simulink model "SW_8"  (R2013b)
settings: Solver=ode45  StartTime=0.0  StopTime=128  RelTol=1e-3
values from neighbouring files (symbols this model uses):
  const_val_lenqs = Nq-1    [confSim.m]    (also in preS_confSim.m)
  g = 1    [confSim.m]
  MiS = -5    [confSim.m]
  MS = 5    [confSim.m]
  nb_counter = ceil(log2(Ns))    [confSim.m]    (also in preS_confSim.m)
  NBitsScoreBus = 10    [confSim.m]    (also in preS_confSim.m)
  Nq = length(qCode)    [confSim.m]    (also in preS_confSim.m)
  Ns = length(sCode)    [confSim.m]    (also in preS_confSim.m)
  qCode = base2dec(q,Base)    [confSim.m]
  sCode = base2dec(s,Base)    [confSim.m]
  SMR_len = Nq*3    [confSim.m]    (also in preS_confSim.m)
libraries: xbsIndex_r4 x1212
(part 5 of 7)

== system SW_8/Subsystem/Subsystem5/P1_HW0 ==
  "reset " : Inport
  M_j-1(n)1 : Inport  Port=2
  MaxValue_j-1 : Inport  Port=3
  EndMaxRAM_j-1 : Inport  Port=4
  EndMaxP_j-1 : Inport  Port=5
  j-1 : Inport  Port=6
  s(n) : Inport  Port=7
  EnIn : Inport  Port=8
  q_j : Inport  Port=9
  AddSub : xbsIndex_r4/AddSub  mode=Addition  use_carryin=off  use_carryout=off  en=off  latency=as0  precision=User Defined  arith_type="Signed  (2's comp)"  n_bits=NBitsCalcInt  bin_pt=0  quantization=Truncate  overflow=Saturate  dbl_ovrd=off  use_behavioral_HDL=off  hw_selection=Fabric  pipelined=off  block_type=addsub
  AddSub1 : xbsIndex_r4/AddSub  mode=Subtraction  use_carryin=off  use_carryout=off  en=off  latency=as0  precision=User Defined  arith_type="Signed  (2's comp)"  n_bits=NBitsCalcInt  bin_pt=0  quantization=Truncate  overflow=Saturate  dbl_ovrd=off  use_behavioral_HDL=off  hw_selection=Fabric  pipelined=off  block_type=addsub
  AddSub2 : xbsIndex_r4/AddSub  mode=Subtraction  use_carryin=off  use_carryout=off  en=off  latency=as0  precision=User Defined  arith_type="Signed  (2's comp)"  n_bits=NBitsCalcInt  bin_pt=0  quantization=Truncate  overflow=Saturate  dbl_ovrd=off  use_behavioral_HDL=off  hw_selection=Fabric  pipelined=off  block_type=addsub
  Constant 0 : xbsIndex_r4/Constant  const=0  gui_display_data_type=Fixed-point  arith_type=Unsigned  n_bits=nb_bool  bin_pt=0  preci_type=Single  exp_width=8  frac_width=24  explicit_period=off  period=1  equ=P=C  opselect=C  inp2=PCIN>>17  opr=+  inp1=P  carry=CIN  dbl_ovrd=off  block_type=constant
  Convert : xbsIndex_r4/Convert  gui_display_data_type=Fixed-point  arith_type=Unsigned  n_bits=nb_bool  bin_pt=0  float_type=Single  exp_bits=8  fraction_bits=24  quantization=Truncate  overflow=Wrap  en=off  latency=c0  dbl_ovrd=off  pipeline=off  block_type=convert
  Convert1 : xbsIndex_r4/Convert  gui_display_data_type=Fixed-point  arith_type=Unsigned  n_bits=k  bin_pt=0  float_type=Single  exp_bits=8  fraction_bits=24  quantization=Truncate  overflow=Wrap  en=off  latency=c0  dbl_ovrd=off  pipeline=off  block_type=convert
  Convert2 : xbsIndex_r4/Convert  gui_display_data_type=Fixed-point  arith_type=Unsigned  n_bits=nb_bool  bin_pt=0  float_type=Single  exp_bits=8  fraction_bits=24  quantization=Truncate  overflow=Wrap  en=off  latency=c0  dbl_ovrd=off  pipeline=off  block_type=convert
  Convert3 : xbsIndex_r4/Convert  gui_display_data_type=Fixed-point  arith_type=Unsigned  n_bits=NBitsCalcInt  bin_pt=0  float_type=Single  exp_bits=8  fraction_bits=24  quantization=Truncate  overflow=Wrap  en=off  latency=c0  dbl_ovrd=off  pipeline=off  block_type=convert
  Convert4 : xbsIndex_r4/Convert  gui_display_data_type=Boolean  arith_type=Boolean  n_bits=1  bin_pt=0  float_type=Single  exp_bits=8  fraction_bits=24  quantization=Truncate  overflow=Wrap  en=off  latency=c0  dbl_ovrd=off  pipeline=off  block_type=convert
  Counter : xbsIndex_r4/Counter  cnt_type=Count Limited  cnt_to=counter_val  operation=Up  start_count=0  cnt_by_val=1  arith_type=Unsigned  n_bits=counter_num_b  bin_pt=0  load_pin=off  rst=on  en=on  explicit_period=on  period=Ts  dbl_ovrd=off  use_behavioral_HDL=off  implementation=Fabric  block_type=counter
  Inverter : xbsIndex_r4/Inverter  en=off  latency=l0  dbl_ovrd=off  block_type=inv
  Inverter1 : xbsIndex_r4/Inverter  en=off  latency=l0  dbl_ovrd=off  block_type=inv
  Inverter2 : xbsIndex_r4/Inverter  en=off  latency=l0  dbl_ovrd=off  block_type=inv
  Logical : xbsIndex_r4/Logical  logical_function=AND  inputs=2  en=off  latency=l0  precision=User Defined  arith_type=Unsigned  n_bits=nb_bool  bin_pt=0  align_bp=on  dbl_ovrd=off  block_type=logical
  MS Match_Score : xbsIndex_r4/Constant  const=MS  gui_display_data_type=Fixed-point  arith_type=Signed (2's comp)  n_bits=NBitsK  bin_pt=0  preci_type=Single  exp_width=8  frac_width=24  explicit_period=on  period=Ts  equ=P=C  opselect=C  inp2=PCIN>>17  opr=+  inp1=P  carry=CIN  dbl_ovrd=off  block_type=constant
  M_j(n-1) : xbsIndex_r4/Register  init=0  rst=on  en=on  dbl_ovrd=off  block_type=register
  Match and Mismtach Score : Subsystem
  Max1 : Subsystem
  MiS MisMatch_Score : xbsIndex_r4/Constant  const=MiS  gui_display_data_type=Fixed-point  arith_type=Signed (2's comp)  n_bits=NBitsK  bin_pt=0  preci_type=Single  exp_width=8  frac_width=24  explicit_period=on  period=Ts  equ=P=C  opselect=C  inp2=PCIN>>17  opr=+  inp1=P  carry=CIN  dbl_ovrd=off  block_type=constant
  Mux1 : xbsIndex_r4/Mux  inputs=2  en=off  latency=mft  precision=User Defined  arith_type=Unsigned  n_bits=counter_num_b  bin_pt=0  quantization=Truncate  overflow=Wrap  dbl_ovrd=off  block_type=mux
  Mux2 : xbsIndex_r4/Mux  inputs=2  en=off  latency=mft  precision=User Defined  arith_type=Unsigned  n_bits=NBitsCalcInt  bin_pt=0  quantization=Truncate  overflow=Wrap  dbl_ovrd=off  block_type=mux
  Mux3 : xbsIndex_r4/Mux  inputs=2  en=off  latency=mft  precision=User Defined  arith_type=Unsigned  n_bits=counter_num_b  bin_pt=0  quantization=Truncate  overflow=Wrap  dbl_ovrd=off  block_type=mux
  Mux4 : xbsIndex_r4/Mux  inputs=2  en=off  latency=mft  precision=User Defined  arith_type=Unsigned  n_bits=nb_lqC  bin_pt=0  quantization=Truncate  overflow=Wrap  dbl_ovrd=off  block_type=mux
  Mux5 : xbsIndex_r4/Mux  inputs=2  en=off  latency=mft  precision=User Defined  arith_type=Unsigned  n_bits=nb_bool  bin_pt=0  quantization=Truncate  overflow=Wrap  dbl_ovrd=off  block_type=mux
  Mux6 : xbsIndex_r4/Mux  inputs=2  en=off  latency=mft  precision=User Defined  arith_type=Unsigned  n_bits=NBitsCalcInt  bin_pt=0  quantization=Truncate  overflow=Wrap  dbl_ovrd=off  block_type=mux
  Mux7 : xbsIndex_r4/Mux  inputs=2  en=off  latency=mft  precision=User Defined  arith_type=Unsigned  n_bits=NBitsCalcInt  bin_pt=0  quantization=Truncate  overflow=Wrap  dbl_ovrd=off  block_type=mux
  Mux8 : xbsIndex_r4/Mux  inputs=2  en=off  latency=mft  precision=User Defined  arith_type=Unsigned  n_bits=k  bin_pt=0  quantization=Truncate  overflow=Wrap  dbl_ovrd=off  block_type=mux
  RM_j-1 : xbsIndex_r4/Register  init=0  rst=on  en=off  dbl_ovrd=off  block_type=register
  RM_j-2 : xbsIndex_r4/Register  init=0  rst=on  en=off  dbl_ovrd=off  block_type=register
  RMax_j : xbsIndex_r4/Register  init=0  rst=on  en=off  dbl_ovrd=off  block_type=register
  RMax_j2 : xbsIndex_r4/Register  init=0  rst=on  en=off  dbl_ovrd=off  block_type=register
  Relational1 : xbsIndex_r4/Relational  mode=a>b  en=off  latency=r0  dbl_ovrd=off  block_type=relational
  Relational2 : xbsIndex_r4/Relational  mode=a>b  en=off  latency=r0  dbl_ovrd=off  block_type=relational
  Relational3 : xbsIndex_r4/Relational  mode=a=b  en=off  latency=r0  dbl_ovrd=off  block_type=relational
  Relational4 : xbsIndex_r4/Relational  mode=a<b  en=off  latency=r0  dbl_ovrd=off  block_type=relational
  "bias " : xbsIndex_r4/Constant  const=1  gui_display_data_type=Fixed-point  arith_type=Signed (2's comp)  n_bits=NBitsScoreBus(1)  bin_pt=0  preci_type=Single  exp_width=8  frac_width=24  explicit_period=off  period=1  equ=P=C  opselect=C  inp2=PCIN>>17  opr=+  inp1=P  carry=CIN  dbl_ovrd=off  block_type=constant
  delay_sync{2,4,9..10} (4 alike) : xbsIndex_r4/Register  init=0  rst=on  en=off  dbl_ovrd=off  block_type=register
  delay_sync8 : xbsIndex_r4/Register  init=0  rst=off  en=off  dbl_ovrd=off  block_type=register
  g Gap_Penalty : xbsIndex_r4/Constant  const=g  gui_display_data_type=Fixed-point  arith_type=Signed (2's comp)  n_bits=NBitsK  bin_pt=0  preci_type=Single  exp_width=8  frac_width=24  explicit_period=on  period=Ts  equ=P=C  opselect=C  inp2=PCIN>>17  opr=+  inp1=P  carry=CIN  dbl_ovrd=off  block_type=constant
  len_q(s) Match_Score1 : xbsIndex_r4/Constant  const=const_val_lenqs  gui_display_data_type=Fixed-point  arith_type=Unsigned  n_bits=const_num_b_lenqs  bin_pt=0  preci_type=Single  exp_width=8  frac_width=24  explicit_period=off  period=1  equ=P=C  opselect=C  inp2=PCIN>>17  opr=+  inp1=P  carry=CIN  dbl_ovrd=off  block_type=constant
  "u+bias " : xbsIndex_r4/AddSub  mode=Addition  use_carryin=off  use_carryout=off  en=off  latency=0  precision=User Defined  arith_type="Signed  (2's comp)"  n_bits=NBitsCalcInt  bin_pt=0  quantization=Truncate  overflow=Saturate  dbl_ovrd=off  use_behavioral_HDL=off  hw_selection=Fabric  pipelined=off  block_type=addsub
  M_j(n) : Outport
  MaxValue : Outport  Port=2
  EndMaxRAM (valor de i) : Outport  Port=3
  EndMaxP (valor de j) : Outport  Port=4
  j : Outport  Port=5
  s(n-1) : Outport  Port=6
  EnOut(n) : Outport  Port=7
  Direction : Outport  Port=8
  wEnd : Outport  Port=9
  TraceBackStart : Outport  Port=10
  out_j : Outport  Port=11
  wires:
  Mux7/1 -> Relational1/1, Mux6/3, M_j(n)/1, M_j(n-1)/1
  Max1/2(value) -> Mux7/2
  Convert3/1 -> Mux7/3
  Convert1/1 -> Mux8/3
  Mux8/1 -> Direction/1
  Inverter2/1 -> Mux8/1
  Inverter1/1 -> Mux7/1
  Logical/1 -> Convert4/1
  Relational3/1 -> Mux5/1, Inverter/1
  j-1/1 -> out_j/1, Relational3/1, "u+bias "/1, Mux4/3
  delay_sync10/1 -> EnOut(n)/1
  delay_sync9/1 -> TraceBackStart/1
  q_j/1 -> Match and Mismtach Score/1(q_j)
  Relational4/1 -> Convert2/1
  Convert2/1 -> Mux5/3
  delay_sync8/1 -> Relational4/2
  Convert/1 -> Relational4/1, delay_sync8/1
  Inverter/1 -> Logical/2
  Constant 0/1 -> Mux5/2
  len_q(s) Match_Score1/1 -> Relational3/2
  Mux4/1 -> EndMaxP (valor de j)/1
  Mux3/1 -> EndMaxRAM (valor de i)/1
  Mux2/1 -> MaxValue/1
  MaxValue_j-1/1 -> Relational2/2, Mux2/2
  EndMaxRAM_j-1/1 -> Mux3/2
  EndMaxP_j-1/1 -> Mux4/2
  delay_sync4/1 -> j/1
  "u+bias "/1 -> delay_sync4/1
  "bias "/1 -> "u+bias "/2
  delay_sync2/1 -> s(n-1)/1
  Relational2/1 -> Mux2/1, Mux3/1, Mux4/1
  RMax_j2/1 -> Mux3/3, Mux1/2
  Mux1/1 -> RMax_j2/1
  RMax_j/1 -> Relational1/2, Relational2/1, Mux2/3, Mux6/2
  Relational1/1 -> Mux1/1, Mux6/1
  Mux6/1 -> RMax_j/1
  Counter/1 -> wEnd/1, Mux1/3
  Match and Mismtach Score/1(MS(q_j,s(n))) -> AddSub/1
  s(n)/1 -> Match and Mismtach Score/2(s(n)), delay_sync2/1  "s(n-1)"
  M_j(n-1)/1 -> AddSub2/1  "RM_j(n-1)"
  AddSub2/1 -> Max1/1((i-1,j))  "(i-1,j)"
  AddSub/1 -> Max1/3((i-1,j-1))  "(i-1,j-1)"
  AddSub1/1 -> Max1/2((i,j-1))  "(i,j-1)"
  g Gap_Penalty/1 -> AddSub2/2, AddSub1/2  "g"
  MiS MisMatch_Score/1 -> Match and Mismtach Score/4(MiS)
  MS Match_Score/1 -> Match and Mismtach Score/3(MS)
  RM_j-1/1 -> AddSub1/1, RM_j-2/1  "M_j-1(n-1)"
  M_j-1(n)1/1 -> RM_j-1/1
  RM_j-2/1 -> AddSub/2  "M_j-1(n-2)"
  Max1/1(ind) -> Mux8/2
  Convert4/1 -> delay_sync10/1
  Mux5/1 -> delay_sync9/1
  "reset "/1 -> delay_sync2/2, RM_j-1/2, delay_sync4/2, delay_sync10/2, delay_sync9/2, RMax_j/2, RMax_j2/2, M_j(n-1)/2, Counter/1, RM_j-2/2
  EnIn/1 -> Inverter2/1, Convert1/1, Inverter1/1, Convert3/1, M_j(n-1)/3, Counter/2, Convert/1, Logical/1

== system SW_8/Subsystem/Subsystem5/_RAM_0 ==
  En(n) : Inport
  RAM_j(n)=i : Inport  Port=2
  D_j(n) : Inport  Port=3
  BT_RAM_j(n)=i : Inport  Port=4
  BTRAMCont : Inport  Port=5
  Concat : xbsIndex_r4/Concat  num_inputs=2  dbl_ovrd=off  block_type=concat
  Logical3 : xbsIndex_r4/Logical  logical_function=AND  inputs=2  en=off  latency=l0  precision=User Defined  arith_type=Unsigned  n_bits=k  bin_pt=0  align_bp=on  dbl_ovrd=off  block_type=logical
  Mux3 : xbsIndex_r4/Mux  inputs=2  en=off  latency=mft  precision=User Defined  arith_type=Unsigned  n_bits=counter_num_b  bin_pt=0  quantization=Truncate  overflow=Wrap  dbl_ovrd=off  block_type=mux
  "RNq " : xbsIndex_r4/Register  init=0  rst=off  en=off  dbl_ovrd=off  block_type=register
  Register : xbsIndex_r4/Register  init=0  rst=off  en=off  dbl_ovrd=off  block_type=register
  Register2 : xbsIndex_r4/Register  init=0  rst=off  en=off  dbl_ovrd=off  block_type=register
  Register4 : xbsIndex_r4/Register  init=0  rst=off  en=off  dbl_ovrd=off  block_type=register
  SWBTRAM1 : xbsIndex_r4/Mux  inputs=2  en=off  latency=mft  precision=User Defined  arith_type=Unsigned  n_bits=nb_bool  bin_pt=0  quantization=Truncate  overflow=Wrap  dbl_ovrd=off  block_type=mux
  Single Port RAM2 : xbsIndex_r4/Single Port RAM  depth=length(sCode)  initVector=zeros(1,length(sCode))  distributed_mem=Distributed memory  write_mode=Read After Write  rst=off  init_reg=0  en=off  latency=Ts  dbl_ovrd=off  optimize=Area  block_type=spram
  D_j(n)1 : Outport
  wires:
  RAM_j(n)=i/1 -> Register2/1
  En(n)/1 -> Register/1
  D_j(n)/1 -> Register4/1
  SWBTRAM1/1 -> Concat/2, Concat/1
  "RNq "/1 -> Logical3/2
  Mux3/1 -> Single Port RAM2/1
  Single Port RAM2/1 -> Logical3/1
  Concat/1 -> "RNq "/1
  Register/1 -> SWBTRAM1/2, Single Port RAM2/3
  BT_RAM_j(n)=i/1 -> Mux3/3
  Register2/1 -> Mux3/2
  BTRAMCont/1 -> Mux3/1, SWBTRAM1/3, SWBTRAM1/1
  Register4/1 -> Single Port RAM2/2
  Logical3/1 -> D_j(n)1/1

== system SW_8/Subsystem/Subsystem5/seq_switch ==
  q_j(n) : Inport
  "Enable " : Inport  Port=2
  "reset " : Inport  Port=3
  Mux5 : xbsIndex_r4/Mux  inputs=2  en=off  latency=mft  precision=User Defined  arith_type=Unsigned  n_bits=k  bin_pt=0  quantization=Truncate  overflow=Wrap  dbl_ovrd=off  block_type=mux
  U>U/z : Subsystem
  delay_sync1 : xbsIndex_r4/Register  init=0  rst=on  en=off  dbl_ovrd=off  block_type=register
  q_j : Outport
  q_j(n-1) : Outport  Port=2
  wires:
  delay_sync1/1 -> Mux5/2
  U>U/z/1(Out1) -> Mux5/1
  Mux5/1 -> delay_sync1/1, q_j/1
  q_j(n)/1 -> Mux5/3, q_j(n-1)/1  "q_j(n-1)"
  "Enable "/1 -> U>U/z/1(In1)
  "reset "/1 -> delay_sync1/2, U>U/z/2(reset)

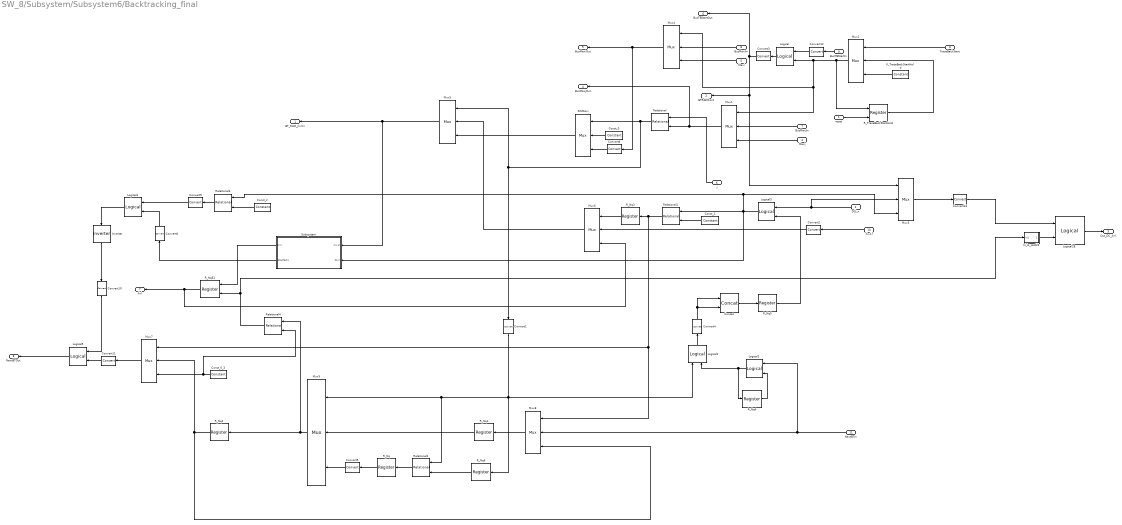
== system SW_8/Subsystem/Subsystem6/Backtracking_final ==
  "reset " : Inport
  "D(j)_n " : Inport  Port=2
  TraceBackStart : Inport  Port=3
  Maxj : Inport  Port=4
  Maxi : Inport  Port=5
  j : Inport  Port=6
  BusMaxjIn : Inport  Port=7
  BusMaxiIn : Inport  Port=8
  BusTBStartIn : Inport  Port=9
  i(n-1) : Inport  Port=10
  NextBTIn : Inport  Port=11
  Concat : xbsIndex_r4/Concat  num_inputs=2  dbl_ovrd=off  block_type=concat
  Const_0 : xbsIndex_r4/Constant  const=0  gui_display_data_type=Fixed-point  arith_type=Unsigned  n_bits=1  bin_pt=0  preci_type=Single  exp_width=8  frac_width=24  explicit_period=on  period=Ts  equ=P=C  opselect=C  inp2=PCIN>>17  opr=+  inp1=P  carry=CIN  dbl_ovrd=off  block_type=constant
  Const_0_3 : xbsIndex_r4/Constant  const=0  gui_display_data_type=Fixed-point  arith_type=Unsigned  n_bits=1  bin_pt=0  preci_type=Single  exp_width=8  frac_width=24  explicit_period=on  period=Ts  equ=P=C  opselect=C  inp2=PCIN>>17  opr=+  inp1=P  carry=CIN  dbl_ovrd=off  block_type=constant
  Const_1 : xbsIndex_r4/Constant  const=1  gui_display_data_type=Fixed-point  arith_type=Unsigned  n_bits=k  bin_pt=0  preci_type=Single  exp_width=8  frac_width=24  explicit_period=on  period=Ts  equ=P=C  opselect=C  inp2=PCIN>>17  opr=+  inp1=P  carry=CIN  dbl_ovrd=off  block_type=constant
  Const_2 : xbsIndex_r4/Constant  const=0  gui_display_data_type=Fixed-point  arith_type=Unsigned  n_bits=k  bin_pt=0  preci_type=Single  exp_width=8  frac_width=24  explicit_period=on  period=Ts  equ=P=C  opselect=C  inp2=PCIN>>17  opr=+  inp1=P  carry=CIN  dbl_ovrd=off  block_type=constant
  Convert1 : xbsIndex_r4/Convert  gui_display_data_type=Fixed-point  arith_type=Unsigned  n_bits=1  bin_pt=0  float_type=Single  exp_bits=8  fraction_bits=24  quantization=Truncate  overflow=Wrap  en=off  latency=c0  dbl_ovrd=off  pipeline=off  block_type=convert
  Convert{5,8..11} (5 alike) : xbsIndex_r4/Convert  gui_display_data_type=Fixed-point  arith_type=Unsigned  n_bits=nb_bool  bin_pt=0  float_type=Single  exp_bits=8  fraction_bits=24  quantization=Truncate  overflow=Wrap  en=off  latency=c0  dbl_ovrd=off  pipeline=off  block_type=convert
  Convert12 : xbsIndex_r4/Convert  gui_display_data_type=Fixed-point  arith_type=Unsigned  n_bits=1  bin_pt=0  float_type=Single  exp_bits=8  fraction_bits=24  quantization=Truncate  overflow=Wrap  en=off  latency=c0  dbl_ovrd=off  pipeline=off  block_type=convert
  Convert13 : xbsIndex_r4/Convert  gui_display_data_type=Fixed-point  arith_type=Unsigned  n_bits=k  bin_pt=0  float_type=Single  exp_bits=8  fraction_bits=24  quantization=Truncate  overflow=Wrap  en=off  latency=0  dbl_ovrd=off  pipeline=off  block_type=convert
  Convert2 : xbsIndex_r4/Convert  gui_display_data_type=Fixed-point  arith_type=Unsigned  n_bits=counter_num_b  bin_pt=0  float_type=Single  exp_bits=8  fraction_bits=24  quantization=Truncate  overflow=Wrap  en=off  latency=c0  dbl_ovrd=off  pipeline=off  block_type=convert
  Convert3 : xbsIndex_r4/Convert  gui_display_data_type=Boolean  arith_type=Boolean  n_bits=1  bin_pt=0  float_type=Single  exp_bits=8  fraction_bits=24  quantization=Truncate  overflow=Wrap  en=off  latency=c0  dbl_ovrd=off  pipeline=off  block_type=convert
  Convert4 : xbsIndex_r4/Convert  gui_display_data_type=Boolean  arith_type=Boolean  n_bits=1  bin_pt=0  float_type=Single  exp_bits=8  fraction_bits=24  quantization=Truncate  overflow=Wrap  en=off  latency=c0  dbl_ovrd=off  pipeline=off  block_type=convert
  Convert6 : xbsIndex_r4/Convert  gui_display_data_type=Fixed-point  arith_type=Unsigned  n_bits=counter_num_b  bin_pt=0  float_type=Single  exp_bits=8  fraction_bits=24  quantization=Truncate  overflow=Wrap  en=off  latency=c0  dbl_ovrd=off  pipeline=off  block_type=convert
  Inverter : xbsIndex_r4/Inverter  en=off  latency=l0  dbl_ovrd=off  block_type=inv
  K_TraceBackStartHold : xbsIndex_r4/Constant  const=1  gui_display_data_type=Fixed-point  arith_type=Unsigned  n_bits=1  bin_pt=0  preci_type=Single  exp_width=8  frac_width=24  explicit_period=on  period=Ts  equ=P=C  opselect=C  inp2=PCIN>>17  opr=+  inp1=P  carry=CIN  dbl_ovrd=off  block_type=constant
  Logical{,1..2,4} (4 alike) : xbsIndex_r4/Logical  logical_function=OR  inputs=2  en=off  latency=l0  precision=User Defined  arith_type=Unsigned  n_bits=nb_bool  bin_pt=0  align_bp=on  dbl_ovrd=off  block_type=logical
  Logical28 : xbsIndex_r4/Logical  logical_function=AND  inputs=2  en=off  latency=l0  precision=User Defined  arith_type=Unsigned  n_bits=k  bin_pt=0  align_bp=on  dbl_ovrd=off  block_type=logical
  Logical3 : xbsIndex_r4/Logical  logical_function=AND  inputs=2  en=off  latency=l0  precision=User Defined  arith_type=Unsigned  n_bits=k  bin_pt=0  align_bp=on  dbl_ovrd=off  block_type=logical
  Logical5 : xbsIndex_r4/Logical  logical_function=AND  inputs=2  en=off  latency=l0  precision=User Defined  arith_type=Unsigned  n_bits=nb_bool  bin_pt=0  align_bp=on  dbl_ovrd=off  block_type=logical
  Mux1 : xbsIndex_r4/Mux  inputs=2  en=off  latency=mft  precision=User Defined  arith_type=Unsigned  n_bits=nb_lqC  bin_pt=0  quantization=Truncate  overflow=Wrap  dbl_ovrd=off  block_type=mux
  Mux2 : xbsIndex_r4/Mux  inputs=2  en=off  latency=mft  precision=User Defined  arith_type=Unsigned  n_bits=nb_bool  bin_pt=0  quantization=Truncate  overflow=Wrap  dbl_ovrd=off  block_type=mux
  Mux3 : xbsIndex_r4/Mux  inputs=2  en=off  latency=mft  precision=User Defined  arith_type=Unsigned  n_bits=k  bin_pt=0  quantization=Truncate  overflow=Wrap  dbl_ovrd=off  block_type=mux
  Mux4 : xbsIndex_r4/Mux  inputs=2  en=off  latency=mft  precision=User Defined  arith_type=Unsigned  n_bits=counter_num_b  bin_pt=0  quantization=Truncate  overflow=Wrap  dbl_ovrd=off  block_type=mux
  Mux5 : xbsIndex_r4/Mux  inputs=2  en=off  latency=mft  precision=User Defined  arith_type=Unsigned  n_bits=counter_num_b  bin_pt=0  quantization=Truncate  overflow=Wrap  dbl_ovrd=off  block_type=mux
  Mux6 : xbsIndex_r4/Mux  inputs=2  en=off  latency=mft  precision=User Defined  arith_type=Unsigned  n_bits=counter_num_b  bin_pt=0  quantization=Truncate  overflow=Wrap  dbl_ovrd=off  block_type=mux
  Mux7 : xbsIndex_r4/Mux  inputs=2  en=off  latency=0  precision=User Defined  arith_type=Unsigned  n_bits=nb_bool  bin_pt=0  quantization=Truncate  overflow=Wrap  dbl_ovrd=off  block_type=mux
  Mux8 : xbsIndex_r4/Mux  inputs=2  en=off  latency=mft  precision=User Defined  arith_type=Unsigned  n_bits=nb_bool  bin_pt=0  quantization=Truncate  overflow=Wrap  dbl_ovrd=off  block_type=mux
  Mux9 : xbsIndex_r4/Mux  inputs=2  en=off  latency=mft  precision=User Defined  arith_type=Unsigned  n_bits=nb_bool  bin_pt=0  quantization=Truncate  overflow=Wrap  dbl_ovrd=off  block_type=mux
  R_Nq{,1..6} (7 alike) : xbsIndex_r4/Register  init=0  rst=off  en=off  dbl_ovrd=off  block_type=register
  R_NqE1 : xbsIndex_r4/Register  init=0  rst=off  en=on  dbl_ovrd=off  block_type=register
  R_TraceBackStartHold : xbsIndex_r4/Register  init=0  rst=on  en=off  dbl_ovrd=off  block_type=register
  Relational : xbsIndex_r4/Relational  mode=a=b  en=off  latency=r0  dbl_ovrd=off  block_type=relational
  Relational1 : xbsIndex_r4/Relational  mode=a=b  en=off  latency=r0  dbl_ovrd=off  block_type=relational
  Relational2 : xbsIndex_r4/Relational  mode=a>b  en=off  latency=r0  dbl_ovrd=off  block_type=relational
  Relational3 : xbsIndex_r4/Relational  mode=a=b  en=off  latency=0  dbl_ovrd=off  block_type=relational
  Relational4 : xbsIndex_r4/Relational  mode=a>b  en=off  latency=r0  dbl_ovrd=off  block_type=relational
  SWMaxi : xbsIndex_r4/Mux  inputs=2  en=off  latency=mft  precision=User Defined  arith_type=Unsigned  n_bits=counter_num_b  bin_pt=0  quantization=Truncate  overflow=Wrap  dbl_ovrd=off  block_type=mux
  Subsystem : Subsystem
  hi_lo_cast22 : Subsystem
  BT_RAM_j(n)=i : Outport
  BTRAMCont : Outport  Port=2
  Out_DC_j(n) : Outport  Port=3
  BusMaxjOut : Outport  Port=4
  BusMaxiOut : Outport  Port=5
  BusTBStartOut : Outport  Port=6
  i(n) : Outport  Port=7
  NextBTOut : Outport  Port=8
  wires:
  Logical28/1 -> Out_DC_j(n)/1
  hi_lo_cast22/1(Out1) -> Logical28/2
  Relational4/1 -> R_NqE1/2, hi_lo_cast22/1(In1)
  Convert13/1 -> Logical28/1
  Convert12/1 -> Logical/1
  Convert11/1 -> Logical5/2
  Convert10/1 -> Logical5/1
  Inverter/1 -> Convert10/1
  Mux7/1 -> Convert11/1
  Logical4/1 -> Inverter/1
  Subsystem/2(StopTBC1) -> Convert8/1
  Convert9/1 -> Logical4/1
  Convert8/1 -> Logical4/2
  Relational3/1 -> Convert9/1
  Const_2/1 -> Relational3/2
  Logical3/1 -> Relational1/1, Mux3/3, Relational3/1, Subsystem/2(D(n))
  Convert3/1 -> Mux3/1, BTRAMCont/1, BusTBStartOut/1
  Logical5/1 -> NextBTOut/1
  Mux4/1 -> Convert6/1, BusMaxiOut/1
  Mux1/1 -> Relational/2, BusMaxjOut/1
  R_NqE1/1 -> Mux6/3, i(n)/1
  Mux5/1 -> Subsystem/1(i(n-1)), BT_RAM_j(n)=i/1
  BusMaxjIn/1 -> Mux1/2
  Maxj/1 -> Mux1/3
  Maxi/1 -> Mux4/3
  TraceBackStart/1 -> Mux2/1
  j/1 -> Relational/1
  BusMaxiIn/1 -> Mux4/2
  BusTBStartIn/1 -> Convert12/1
  NextBTIn/1 -> Logical1/1, Mux8/2
  i(n-1)/1 -> Convert2/1
  "D(j)_n "/1 -> Logical3/1, Mux3/2
  Mux3/1 -> Convert13/1
  Mux2/1 -> R_TraceBackStartHold/1, Logical/2, Mux1/1, Mux4/1
  Convert6/1 -> SWMaxi/3
  SWMaxi/1 -> Mux5/3
  Mux6/1 -> Mux5/2
  Convert5/1 -> Mux9/3
  Mux9/1 -> Relational4/1, R_Nq2/1
  Convert2/1 -> Mux6/2
  Convert1/1 -> Mux9/1, Relational2/1, R_Nq6/1, Logical2/1
  Relational/1 -> SWMaxi/1, Convert1/1, Mux5/1
  Convert4/1 -> Concat/2, Concat/1
  R_Nq6/1 -> Relational2/2
  R_Nq1/1 -> Mux9/2
  R_Nq/1 -> Convert5/1
  R_TraceBackStartHold/1 -> Mux2/2
  Const_0/1 -> SWMaxi/2
  Mux8/1 -> R_Nq1/1
  Relational2/1 -> R_Nq/1
  R_Nq2/1 -> Mux8/3, Mux7/2
  Const_1/1 -> Relational1/2
  Relational1/1 -> R_Nq3/1, Mux7/1, Mux8/1
  R_Nq5/1 -> Logical3/2
  R_Nq3/1 -> Mux6/1
  Logical1/1 -> R_Nq4/1, Logical2/2
  Concat/1 -> R_Nq5/1
  Subsystem/1(i(n)) -> R_NqE1/1
  Const_0_3/1 -> Mux7/3, Relational4/2
  Logical/1 -> Convert3/1
  R_Nq4/1 -> Logical1/2
  K_TraceBackStartHold/1 -> Mux2/3
  Logical2/1 -> Convert4/1
  "reset "/1 -> R_TraceBackStartHold/2

== system SW_8/Subsystem/Subsystem6/P1_HW0 ==
  "reset " : Inport
  M_j-1(n)1 : Inport  Port=2
  MaxValue_j-1 : Inport  Port=3
  EndMaxRAM_j-1 : Inport  Port=4
  EndMaxP_j-1 : Inport  Port=5
  j-1 : Inport  Port=6
  s(n) : Inport  Port=7
  EnIn : Inport  Port=8
  q_j : Inport  Port=9
  AddSub : xbsIndex_r4/AddSub  mode=Addition  use_carryin=off  use_carryout=off  en=off  latency=as0  precision=User Defined  arith_type="Signed  (2's comp)"  n_bits=NBitsCalcInt  bin_pt=0  quantization=Truncate  overflow=Saturate  dbl_ovrd=off  use_behavioral_HDL=off  hw_selection=Fabric  pipelined=off  block_type=addsub
  AddSub1 : xbsIndex_r4/AddSub  mode=Subtraction  use_carryin=off  use_carryout=off  en=off  latency=as0  precision=User Defined  arith_type="Signed  (2's comp)"  n_bits=NBitsCalcInt  bin_pt=0  quantization=Truncate  overflow=Saturate  dbl_ovrd=off  use_behavioral_HDL=off  hw_selection=Fabric  pipelined=off  block_type=addsub
  AddSub2 : xbsIndex_r4/AddSub  mode=Subtraction  use_carryin=off  use_carryout=off  en=off  latency=as0  precision=User Defined  arith_type="Signed  (2's comp)"  n_bits=NBitsCalcInt  bin_pt=0  quantization=Truncate  overflow=Saturate  dbl_ovrd=off  use_behavioral_HDL=off  hw_selection=Fabric  pipelined=off  block_type=addsub
  Constant 0 : xbsIndex_r4/Constant  const=0  gui_display_data_type=Fixed-point  arith_type=Unsigned  n_bits=nb_bool  bin_pt=0  preci_type=Single  exp_width=8  frac_width=24  explicit_period=off  period=1  equ=P=C  opselect=C  inp2=PCIN>>17  opr=+  inp1=P  carry=CIN  dbl_ovrd=off  block_type=constant
  Convert : xbsIndex_r4/Convert  gui_display_data_type=Fixed-point  arith_type=Unsigned  n_bits=nb_bool  bin_pt=0  float_type=Single  exp_bits=8  fraction_bits=24  quantization=Truncate  overflow=Wrap  en=off  latency=c0  dbl_ovrd=off  pipeline=off  block_type=convert
  Convert1 : xbsIndex_r4/Convert  gui_display_data_type=Fixed-point  arith_type=Unsigned  n_bits=k  bin_pt=0  float_type=Single  exp_bits=8  fraction_bits=24  quantization=Truncate  overflow=Wrap  en=off  latency=c0  dbl_ovrd=off  pipeline=off  block_type=convert
  Convert2 : xbsIndex_r4/Convert  gui_display_data_type=Fixed-point  arith_type=Unsigned  n_bits=nb_bool  bin_pt=0  float_type=Single  exp_bits=8  fraction_bits=24  quantization=Truncate  overflow=Wrap  en=off  latency=c0  dbl_ovrd=off  pipeline=off  block_type=convert
  Convert3 : xbsIndex_r4/Convert  gui_display_data_type=Fixed-point  arith_type=Unsigned  n_bits=NBitsCalcInt  bin_pt=0  float_type=Single  exp_bits=8  fraction_bits=24  quantization=Truncate  overflow=Wrap  en=off  latency=c0  dbl_ovrd=off  pipeline=off  block_type=convert
  Convert4 : xbsIndex_r4/Convert  gui_display_data_type=Boolean  arith_type=Boolean  n_bits=1  bin_pt=0  float_type=Single  exp_bits=8  fraction_bits=24  quantization=Truncate  overflow=Wrap  en=off  latency=c0  dbl_ovrd=off  pipeline=off  block_type=convert
  Counter : xbsIndex_r4/Counter  cnt_type=Count Limited  cnt_to=counter_val  operation=Up  start_count=0  cnt_by_val=1  arith_type=Unsigned  n_bits=counter_num_b  bin_pt=0  load_pin=off  rst=on  en=on  explicit_period=on  period=Ts  dbl_ovrd=off  use_behavioral_HDL=off  implementation=Fabric  block_type=counter
  Inverter : xbsIndex_r4/Inverter  en=off  latency=l0  dbl_ovrd=off  block_type=inv
  Inverter1 : xbsIndex_r4/Inverter  en=off  latency=l0  dbl_ovrd=off  block_type=inv
  Inverter2 : xbsIndex_r4/Inverter  en=off  latency=l0  dbl_ovrd=off  block_type=inv
  Logical : xbsIndex_r4/Logical  logical_function=AND  inputs=2  en=off  latency=l0  precision=User Defined  arith_type=Unsigned  n_bits=nb_bool  bin_pt=0  align_bp=on  dbl_ovrd=off  block_type=logical
  MS Match_Score : xbsIndex_r4/Constant  const=MS  gui_display_data_type=Fixed-point  arith_type=Signed (2's comp)  n_bits=NBitsK  bin_pt=0  preci_type=Single  exp_width=8  frac_width=24  explicit_period=on  period=Ts  equ=P=C  opselect=C  inp2=PCIN>>17  opr=+  inp1=P  carry=CIN  dbl_ovrd=off  block_type=constant
  M_j(n-1) : xbsIndex_r4/Register  init=0  rst=on  en=on  dbl_ovrd=off  block_type=register
  Match and Mismtach Score : Subsystem
  Max1 : Subsystem
  MiS MisMatch_Score : xbsIndex_r4/Constant  const=MiS  gui_display_data_type=Fixed-point  arith_type=Signed (2's comp)  n_bits=NBitsK  bin_pt=0  preci_type=Single  exp_width=8  frac_width=24  explicit_period=on  period=Ts  equ=P=C  opselect=C  inp2=PCIN>>17  opr=+  inp1=P  carry=CIN  dbl_ovrd=off  block_type=constant
  Mux1 : xbsIndex_r4/Mux  inputs=2  en=off  latency=mft  precision=User Defined  arith_type=Unsigned  n_bits=counter_num_b  bin_pt=0  quantization=Truncate  overflow=Wrap  dbl_ovrd=off  block_type=mux
  Mux2 : xbsIndex_r4/Mux  inputs=2  en=off  latency=mft  precision=User Defined  arith_type=Unsigned  n_bits=NBitsCalcInt  bin_pt=0  quantization=Truncate  overflow=Wrap  dbl_ovrd=off  block_type=mux
  Mux3 : xbsIndex_r4/Mux  inputs=2  en=off  latency=mft  precision=User Defined  arith_type=Unsigned  n_bits=counter_num_b  bin_pt=0  quantization=Truncate  overflow=Wrap  dbl_ovrd=off  block_type=mux
  Mux4 : xbsIndex_r4/Mux  inputs=2  en=off  latency=mft  precision=User Defined  arith_type=Unsigned  n_bits=nb_lqC  bin_pt=0  quantization=Truncate  overflow=Wrap  dbl_ovrd=off  block_type=mux
  Mux5 : xbsIndex_r4/Mux  inputs=2  en=off  latency=mft  precision=User Defined  arith_type=Unsigned  n_bits=nb_bool  bin_pt=0  quantization=Truncate  overflow=Wrap  dbl_ovrd=off  block_type=mux
  Mux6 : xbsIndex_r4/Mux  inputs=2  en=off  latency=mft  precision=User Defined  arith_type=Unsigned  n_bits=NBitsCalcInt  bin_pt=0  quantization=Truncate  overflow=Wrap  dbl_ovrd=off  block_type=mux
  Mux7 : xbsIndex_r4/Mux  inputs=2  en=off  latency=mft  precision=User Defined  arith_type=Unsigned  n_bits=NBitsCalcInt  bin_pt=0  quantization=Truncate  overflow=Wrap  dbl_ovrd=off  block_type=mux
  Mux8 : xbsIndex_r4/Mux  inputs=2  en=off  latency=mft  precision=User Defined  arith_type=Unsigned  n_bits=k  bin_pt=0  quantization=Truncate  overflow=Wrap  dbl_ovrd=off  block_type=mux
  RM_j-1 : xbsIndex_r4/Register  init=0  rst=on  en=off  dbl_ovrd=off  block_type=register
  RM_j-2 : xbsIndex_r4/Register  init=0  rst=on  en=off  dbl_ovrd=off  block_type=register
  RMax_j : xbsIndex_r4/Register  init=0  rst=on  en=off  dbl_ovrd=off  block_type=register
  RMax_j2 : xbsIndex_r4/Register  init=0  rst=on  en=off  dbl_ovrd=off  block_type=register
  Relational1 : xbsIndex_r4/Relational  mode=a>b  en=off  latency=r0  dbl_ovrd=off  block_type=relational
  Relational2 : xbsIndex_r4/Relational  mode=a>b  en=off  latency=r0  dbl_ovrd=off  block_type=relational
  Relational3 : xbsIndex_r4/Relational  mode=a=b  en=off  latency=r0  dbl_ovrd=off  block_type=relational
  Relational4 : xbsIndex_r4/Relational  mode=a<b  en=off  latency=r0  dbl_ovrd=off  block_type=relational
  "bias " : xbsIndex_r4/Constant  const=1  gui_display_data_type=Fixed-point  arith_type=Signed (2's comp)  n_bits=NBitsScoreBus(1)  bin_pt=0  preci_type=Single  exp_width=8  frac_width=24  explicit_period=off  period=1  equ=P=C  opselect=C  inp2=PCIN>>17  opr=+  inp1=P  carry=CIN  dbl_ovrd=off  block_type=constant
  delay_sync{2,4,9..10} (4 alike) : xbsIndex_r4/Register  init=0  rst=on  en=off  dbl_ovrd=off  block_type=register
  delay_sync8 : xbsIndex_r4/Register  init=0  rst=off  en=off  dbl_ovrd=off  block_type=register
  g Gap_Penalty : xbsIndex_r4/Constant  const=g  gui_display_data_type=Fixed-point  arith_type=Signed (2's comp)  n_bits=NBitsK  bin_pt=0  preci_type=Single  exp_width=8  frac_width=24  explicit_period=on  period=Ts  equ=P=C  opselect=C  inp2=PCIN>>17  opr=+  inp1=P  carry=CIN  dbl_ovrd=off  block_type=constant
  len_q(s) Match_Score1 : xbsIndex_r4/Constant  const=const_val_lenqs  gui_display_data_type=Fixed-point  arith_type=Unsigned  n_bits=const_num_b_lenqs  bin_pt=0  preci_type=Single  exp_width=8  frac_width=24  explicit_period=off  period=1  equ=P=C  opselect=C  inp2=PCIN>>17  opr=+  inp1=P  carry=CIN  dbl_ovrd=off  block_type=constant
  "u+bias " : xbsIndex_r4/AddSub  mode=Addition  use_carryin=off  use_carryout=off  en=off  latency=0  precision=User Defined  arith_type="Signed  (2's comp)"  n_bits=NBitsCalcInt  bin_pt=0  quantization=Truncate  overflow=Saturate  dbl_ovrd=off  use_behavioral_HDL=off  hw_selection=Fabric  pipelined=off  block_type=addsub
  M_j(n) : Outport
  MaxValue : Outport  Port=2
  EndMaxRAM (valor de i) : Outport  Port=3
  EndMaxP (valor de j) : Outport  Port=4
  j : Outport  Port=5
  s(n-1) : Outport  Port=6
  EnOut(n) : Outport  Port=7
  Direction : Outport  Port=8
  wEnd : Outport  Port=9
  TraceBackStart : Outport  Port=10
  out_j : Outport  Port=11
  wires:
  Mux7/1 -> Relational1/1, Mux6/3, M_j(n)/1, M_j(n-1)/1
  Max1/2(value) -> Mux7/2
  Convert3/1 -> Mux7/3
  Convert1/1 -> Mux8/3
  Mux8/1 -> Direction/1
  Inverter2/1 -> Mux8/1
  Inverter1/1 -> Mux7/1
  Logical/1 -> Convert4/1
  Relational3/1 -> Mux5/1, Inverter/1
  j-1/1 -> out_j/1, Relational3/1, "u+bias "/1, Mux4/3
  delay_sync10/1 -> EnOut(n)/1
  delay_sync9/1 -> TraceBackStart/1
  q_j/1 -> Match and Mismtach Score/1(q_j)
  Relational4/1 -> Convert2/1
  Convert2/1 -> Mux5/3
  delay_sync8/1 -> Relational4/2
  Convert/1 -> Relational4/1, delay_sync8/1
  Inverter/1 -> Logical/2
  Constant 0/1 -> Mux5/2
  len_q(s) Match_Score1/1 -> Relational3/2
  Mux4/1 -> EndMaxP (valor de j)/1
  Mux3/1 -> EndMaxRAM (valor de i)/1
  Mux2/1 -> MaxValue/1
  MaxValue_j-1/1 -> Relational2/2, Mux2/2
  EndMaxRAM_j-1/1 -> Mux3/2
  EndMaxP_j-1/1 -> Mux4/2
  delay_sync4/1 -> j/1
  "u+bias "/1 -> delay_sync4/1
  "bias "/1 -> "u+bias "/2
  delay_sync2/1 -> s(n-1)/1
  Relational2/1 -> Mux2/1, Mux3/1, Mux4/1
  RMax_j2/1 -> Mux3/3, Mux1/2
  Mux1/1 -> RMax_j2/1
  RMax_j/1 -> Relational1/2, Relational2/1, Mux2/3, Mux6/2
  Relational1/1 -> Mux1/1, Mux6/1
  Mux6/1 -> RMax_j/1
  Counter/1 -> wEnd/1, Mux1/3
  Match and Mismtach Score/1(MS(q_j,s(n))) -> AddSub/1
  s(n)/1 -> Match and Mismtach Score/2(s(n)), delay_sync2/1  "s(n-1)"
  M_j(n-1)/1 -> AddSub2/1  "RM_j(n-1)"
  AddSub2/1 -> Max1/1((i-1,j))  "(i-1,j)"
  AddSub/1 -> Max1/3((i-1,j-1))  "(i-1,j-1)"
  AddSub1/1 -> Max1/2((i,j-1))  "(i,j-1)"
  g Gap_Penalty/1 -> AddSub2/2, AddSub1/2  "g"
  MiS MisMatch_Score/1 -> Match and Mismtach Score/4(MiS)
  MS Match_Score/1 -> Match and Mismtach Score/3(MS)
  RM_j-1/1 -> AddSub1/1, RM_j-2/1  "M_j-1(n-1)"
  M_j-1(n)1/1 -> RM_j-1/1
  RM_j-2/1 -> AddSub/2  "M_j-1(n-2)"
  Max1/1(ind) -> Mux8/2
  Convert4/1 -> delay_sync10/1
  Mux5/1 -> delay_sync9/1
  "reset "/1 -> delay_sync2/2, RM_j-1/2, delay_sync4/2, delay_sync10/2, delay_sync9/2, RMax_j/2, RMax_j2/2, M_j(n-1)/2, Counter/1, RM_j-2/2
  EnIn/1 -> Inverter2/1, Convert1/1, Inverter1/1, Convert3/1, M_j(n-1)/3, Counter/2, Convert/1, Logical/1

== system SW_8/Subsystem/Subsystem6/_RAM_0 ==
  En(n) : Inport
  RAM_j(n)=i : Inport  Port=2
  D_j(n) : Inport  Port=3
  BT_RAM_j(n)=i : Inport  Port=4
  BTRAMCont : Inport  Port=5
  Concat : xbsIndex_r4/Concat  num_inputs=2  dbl_ovrd=off  block_type=concat
  Logical3 : xbsIndex_r4/Logical  logical_function=AND  inputs=2  en=off  latency=l0  precision=User Defined  arith_type=Unsigned  n_bits=k  bin_pt=0  align_bp=on  dbl_ovrd=off  block_type=logical
  Mux3 : xbsIndex_r4/Mux  inputs=2  en=off  latency=mft  precision=User Defined  arith_type=Unsigned  n_bits=counter_num_b  bin_pt=0  quantization=Truncate  overflow=Wrap  dbl_ovrd=off  block_type=mux
  "RNq " : xbsIndex_r4/Register  init=0  rst=off  en=off  dbl_ovrd=off  block_type=register
  Register : xbsIndex_r4/Register  init=0  rst=off  en=off  dbl_ovrd=off  block_type=register
  Register2 : xbsIndex_r4/Register  init=0  rst=off  en=off  dbl_ovrd=off  block_type=register
  Register4 : xbsIndex_r4/Register  init=0  rst=off  en=off  dbl_ovrd=off  block_type=register
  SWBTRAM1 : xbsIndex_r4/Mux  inputs=2  en=off  latency=mft  precision=User Defined  arith_type=Unsigned  n_bits=nb_bool  bin_pt=0  quantization=Truncate  overflow=Wrap  dbl_ovrd=off  block_type=mux
  Single Port RAM2 : xbsIndex_r4/Single Port RAM  depth=length(sCode)  initVector=zeros(1,length(sCode))  distributed_mem=Distributed memory  write_mode=Read After Write  rst=off  init_reg=0  en=off  latency=Ts  dbl_ovrd=off  optimize=Area  block_type=spram
  D_j(n)1 : Outport
  wires:
  RAM_j(n)=i/1 -> Register2/1
  En(n)/1 -> Register/1
  D_j(n)/1 -> Register4/1
  SWBTRAM1/1 -> Concat/2, Concat/1
  "RNq "/1 -> Logical3/2
  Mux3/1 -> Single Port RAM2/1
  Single Port RAM2/1 -> Logical3/1
  Concat/1 -> "RNq "/1
  Register/1 -> SWBTRAM1/2, Single Port RAM2/3
  BT_RAM_j(n)=i/1 -> Mux3/3
  Register2/1 -> Mux3/2
  BTRAMCont/1 -> Mux3/1, SWBTRAM1/3, SWBTRAM1/1
  Register4/1 -> Single Port RAM2/2
  Logical3/1 -> D_j(n)1/1

== system SW_8/Subsystem/Subsystem6/seq_switch ==
  q_j(n) : Inport
  "Enable " : Inport  Port=2
  "reset " : Inport  Port=3
  Mux5 : xbsIndex_r4/Mux  inputs=2  en=off  latency=mft  precision=User Defined  arith_type=Unsigned  n_bits=k  bin_pt=0  quantization=Truncate  overflow=Wrap  dbl_ovrd=off  block_type=mux
  U>U/z : Subsystem
  delay_sync1 : xbsIndex_r4/Register  init=0  rst=on  en=off  dbl_ovrd=off  block_type=register
  q_j : Outport
  q_j(n-1) : Outport  Port=2
  wires:
  delay_sync1/1 -> Mux5/2
  U>U/z/1(Out1) -> Mux5/1
  Mux5/1 -> delay_sync1/1, q_j/1
  q_j(n)/1 -> Mux5/3, q_j(n-1)/1  "q_j(n-1)"
  "Enable "/1 -> U>U/z/1(In1)
  "reset "/1 -> delay_sync1/2, U>U/z/2(reset)

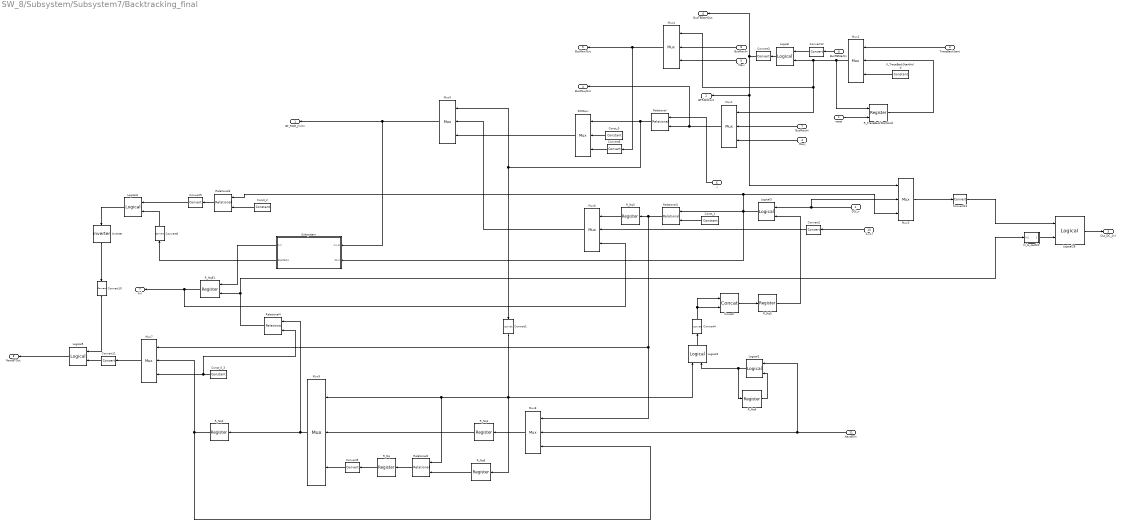
== system SW_8/Subsystem/Subsystem7/Backtracking_final ==
  "reset " : Inport
  "D(j)_n " : Inport  Port=2
  TraceBackStart : Inport  Port=3
  Maxj : Inport  Port=4
  Maxi : Inport  Port=5
  j : Inport  Port=6
  BusMaxjIn : Inport  Port=7
  BusMaxiIn : Inport  Port=8
  BusTBStartIn : Inport  Port=9
  i(n-1) : Inport  Port=10
  NextBTIn : Inport  Port=11
  Concat : xbsIndex_r4/Concat  num_inputs=2  dbl_ovrd=off  block_type=concat
  Const_0 : xbsIndex_r4/Constant  const=0  gui_display_data_type=Fixed-point  arith_type=Unsigned  n_bits=1  bin_pt=0  preci_type=Single  exp_width=8  frac_width=24  explicit_period=on  period=Ts  equ=P=C  opselect=C  inp2=PCIN>>17  opr=+  inp1=P  carry=CIN  dbl_ovrd=off  block_type=constant
  Const_0_3 : xbsIndex_r4/Constant  const=0  gui_display_data_type=Fixed-point  arith_type=Unsigned  n_bits=1  bin_pt=0  preci_type=Single  exp_width=8  frac_width=24  explicit_period=on  period=Ts  equ=P=C  opselect=C  inp2=PCIN>>17  opr=+  inp1=P  carry=CIN  dbl_ovrd=off  block_type=constant
  Const_1 : xbsIndex_r4/Constant  const=1  gui_display_data_type=Fixed-point  arith_type=Unsigned  n_bits=k  bin_pt=0  preci_type=Single  exp_width=8  frac_width=24  explicit_period=on  period=Ts  equ=P=C  opselect=C  inp2=PCIN>>17  opr=+  inp1=P  carry=CIN  dbl_ovrd=off  block_type=constant
  Const_2 : xbsIndex_r4/Constant  const=0  gui_display_data_type=Fixed-point  arith_type=Unsigned  n_bits=k  bin_pt=0  preci_type=Single  exp_width=8  frac_width=24  explicit_period=on  period=Ts  equ=P=C  opselect=C  inp2=PCIN>>17  opr=+  inp1=P  carry=CIN  dbl_ovrd=off  block_type=constant
  Convert1 : xbsIndex_r4/Convert  gui_display_data_type=Fixed-point  arith_type=Unsigned  n_bits=1  bin_pt=0  float_type=Single  exp_bits=8  fraction_bits=24  quantization=Truncate  overflow=Wrap  en=off  latency=c0  dbl_ovrd=off  pipeline=off  block_type=convert
  Convert{5,8..11} (5 alike) : xbsIndex_r4/Convert  gui_display_data_type=Fixed-point  arith_type=Unsigned  n_bits=nb_bool  bin_pt=0  float_type=Single  exp_bits=8  fraction_bits=24  quantization=Truncate  overflow=Wrap  en=off  latency=c0  dbl_ovrd=off  pipeline=off  block_type=convert
  Convert12 : xbsIndex_r4/Convert  gui_display_data_type=Fixed-point  arith_type=Unsigned  n_bits=1  bin_pt=0  float_type=Single  exp_bits=8  fraction_bits=24  quantization=Truncate  overflow=Wrap  en=off  latency=c0  dbl_ovrd=off  pipeline=off  block_type=convert
  Convert13 : xbsIndex_r4/Convert  gui_display_data_type=Fixed-point  arith_type=Unsigned  n_bits=k  bin_pt=0  float_type=Single  exp_bits=8  fraction_bits=24  quantization=Truncate  overflow=Wrap  en=off  latency=0  dbl_ovrd=off  pipeline=off  block_type=convert
  Convert2 : xbsIndex_r4/Convert  gui_display_data_type=Fixed-point  arith_type=Unsigned  n_bits=counter_num_b  bin_pt=0  float_type=Single  exp_bits=8  fraction_bits=24  quantization=Truncate  overflow=Wrap  en=off  latency=c0  dbl_ovrd=off  pipeline=off  block_type=convert
  Convert3 : xbsIndex_r4/Convert  gui_display_data_type=Boolean  arith_type=Boolean  n_bits=1  bin_pt=0  float_type=Single  exp_bits=8  fraction_bits=24  quantization=Truncate  overflow=Wrap  en=off  latency=c0  dbl_ovrd=off  pipeline=off  block_type=convert
  Convert4 : xbsIndex_r4/Convert  gui_display_data_type=Boolean  arith_type=Boolean  n_bits=1  bin_pt=0  float_type=Single  exp_bits=8  fraction_bits=24  quantization=Truncate  overflow=Wrap  en=off  latency=c0  dbl_ovrd=off  pipeline=off  block_type=convert
  Convert6 : xbsIndex_r4/Convert  gui_display_data_type=Fixed-point  arith_type=Unsigned  n_bits=counter_num_b  bin_pt=0  float_type=Single  exp_bits=8  fraction_bits=24  quantization=Truncate  overflow=Wrap  en=off  latency=c0  dbl_ovrd=off  pipeline=off  block_type=convert
  Inverter : xbsIndex_r4/Inverter  en=off  latency=l0  dbl_ovrd=off  block_type=inv
  K_TraceBackStartHold : xbsIndex_r4/Constant  const=1  gui_display_data_type=Fixed-point  arith_type=Unsigned  n_bits=1  bin_pt=0  preci_type=Single  exp_width=8  frac_width=24  explicit_period=on  period=Ts  equ=P=C  opselect=C  inp2=PCIN>>17  opr=+  inp1=P  carry=CIN  dbl_ovrd=off  block_type=constant
  Logical{,1..2,4} (4 alike) : xbsIndex_r4/Logical  logical_function=OR  inputs=2  en=off  latency=l0  precision=User Defined  arith_type=Unsigned  n_bits=nb_bool  bin_pt=0  align_bp=on  dbl_ovrd=off  block_type=logical
  Logical28 : xbsIndex_r4/Logical  logical_function=AND  inputs=2  en=off  latency=l0  precision=User Defined  arith_type=Unsigned  n_bits=k  bin_pt=0  align_bp=on  dbl_ovrd=off  block_type=logical
  Logical3 : xbsIndex_r4/Logical  logical_function=AND  inputs=2  en=off  latency=l0  precision=User Defined  arith_type=Unsigned  n_bits=k  bin_pt=0  align_bp=on  dbl_ovrd=off  block_type=logical
  Logical5 : xbsIndex_r4/Logical  logical_function=AND  inputs=2  en=off  latency=l0  precision=User Defined  arith_type=Unsigned  n_bits=nb_bool  bin_pt=0  align_bp=on  dbl_ovrd=off  block_type=logical
  Mux1 : xbsIndex_r4/Mux  inputs=2  en=off  latency=mft  precision=User Defined  arith_type=Unsigned  n_bits=nb_lqC  bin_pt=0  quantization=Truncate  overflow=Wrap  dbl_ovrd=off  block_type=mux
  Mux2 : xbsIndex_r4/Mux  inputs=2  en=off  latency=mft  precision=User Defined  arith_type=Unsigned  n_bits=nb_bool  bin_pt=0  quantization=Truncate  overflow=Wrap  dbl_ovrd=off  block_type=mux
  Mux3 : xbsIndex_r4/Mux  inputs=2  en=off  latency=mft  precision=User Defined  arith_type=Unsigned  n_bits=k  bin_pt=0  quantization=Truncate  overflow=Wrap  dbl_ovrd=off  block_type=mux
  Mux4 : xbsIndex_r4/Mux  inputs=2  en=off  latency=mft  precision=User Defined  arith_type=Unsigned  n_bits=counter_num_b  bin_pt=0  quantization=Truncate  overflow=Wrap  dbl_ovrd=off  block_type=mux
  Mux5 : xbsIndex_r4/Mux  inputs=2  en=off  latency=mft  precision=User Defined  arith_type=Unsigned  n_bits=counter_num_b  bin_pt=0  quantization=Truncate  overflow=Wrap  dbl_ovrd=off  block_type=mux
  Mux6 : xbsIndex_r4/Mux  inputs=2  en=off  latency=mft  precision=User Defined  arith_type=Unsigned  n_bits=counter_num_b  bin_pt=0  quantization=Truncate  overflow=Wrap  dbl_ovrd=off  block_type=mux
  Mux7 : xbsIndex_r4/Mux  inputs=2  en=off  latency=0  precision=User Defined  arith_type=Unsigned  n_bits=nb_bool  bin_pt=0  quantization=Truncate  overflow=Wrap  dbl_ovrd=off  block_type=mux
  Mux8 : xbsIndex_r4/Mux  inputs=2  en=off  latency=mft  precision=User Defined  arith_type=Unsigned  n_bits=nb_bool  bin_pt=0  quantization=Truncate  overflow=Wrap  dbl_ovrd=off  block_type=mux
  Mux9 : xbsIndex_r4/Mux  inputs=2  en=off  latency=mft  precision=User Defined  arith_type=Unsigned  n_bits=nb_bool  bin_pt=0  quantization=Truncate  overflow=Wrap  dbl_ovrd=off  block_type=mux
  R_Nq{,1..6} (7 alike) : xbsIndex_r4/Register  init=0  rst=off  en=off  dbl_ovrd=off  block_type=register
  R_NqE1 : xbsIndex_r4/Register  init=0  rst=off  en=on  dbl_ovrd=off  block_type=register
  R_TraceBackStartHold : xbsIndex_r4/Register  init=0  rst=on  en=off  dbl_ovrd=off  block_type=register
  Relational : xbsIndex_r4/Relational  mode=a=b  en=off  latency=r0  dbl_ovrd=off  block_type=relational
  Relational1 : xbsIndex_r4/Relational  mode=a=b  en=off  latency=r0  dbl_ovrd=off  block_type=relational
  Relational2 : xbsIndex_r4/Relational  mode=a>b  en=off  latency=r0  dbl_ovrd=off  block_type=relational
  Relational3 : xbsIndex_r4/Relational  mode=a=b  en=off  latency=0  dbl_ovrd=off  block_type=relational
  Relational4 : xbsIndex_r4/Relational  mode=a>b  en=off  latency=r0  dbl_ovrd=off  block_type=relational
  SWMaxi : xbsIndex_r4/Mux  inputs=2  en=off  latency=mft  precision=User Defined  arith_type=Unsigned  n_bits=counter_num_b  bin_pt=0  quantization=Truncate  overflow=Wrap  dbl_ovrd=off  block_type=mux
  Subsystem : Subsystem
  hi_lo_cast22 : Subsystem
  BT_RAM_j(n)=i : Outport
  BTRAMCont : Outport  Port=2
  Out_DC_j(n) : Outport  Port=3
  BusMaxjOut : Outport  Port=4
  BusMaxiOut : Outport  Port=5
  BusTBStartOut : Outport  Port=6
  i(n) : Outport  Port=7
  NextBTOut : Outport  Port=8
  wires:
  Logical28/1 -> Out_DC_j(n)/1
  hi_lo_cast22/1(Out1) -> Logical28/2
  Relational4/1 -> R_NqE1/2, hi_lo_cast22/1(In1)
  Convert13/1 -> Logical28/1
  Convert12/1 -> Logical/1
  Convert11/1 -> Logical5/2
  Convert10/1 -> Logical5/1
  Inverter/1 -> Convert10/1
  Mux7/1 -> Convert11/1
  Logical4/1 -> Inverter/1
  Subsystem/2(StopTBC1) -> Convert8/1
  Convert9/1 -> Logical4/1
  Convert8/1 -> Logical4/2
  Relational3/1 -> Convert9/1
  Const_2/1 -> Relational3/2
  Logical3/1 -> Relational1/1, Mux3/3, Relational3/1, Subsystem/2(D(n))
  Convert3/1 -> Mux3/1, BTRAMCont/1, BusTBStartOut/1
  Logical5/1 -> NextBTOut/1
  Mux4/1 -> Convert6/1, BusMaxiOut/1
  Mux1/1 -> Relational/2, BusMaxjOut/1
  R_NqE1/1 -> Mux6/3, i(n)/1
  Mux5/1 -> Subsystem/1(i(n-1)), BT_RAM_j(n)=i/1
  BusMaxjIn/1 -> Mux1/2
  Maxj/1 -> Mux1/3
  Maxi/1 -> Mux4/3
  TraceBackStart/1 -> Mux2/1
  j/1 -> Relational/1
  BusMaxiIn/1 -> Mux4/2
  BusTBStartIn/1 -> Convert12/1
  NextBTIn/1 -> Logical1/1, Mux8/2
  i(n-1)/1 -> Convert2/1
  "D(j)_n "/1 -> Logical3/1, Mux3/2
  Mux3/1 -> Convert13/1
  Mux2/1 -> R_TraceBackStartHold/1, Logical/2, Mux1/1, Mux4/1
  Convert6/1 -> SWMaxi/3
  SWMaxi/1 -> Mux5/3
  Mux6/1 -> Mux5/2
  Convert5/1 -> Mux9/3
  Mux9/1 -> Relational4/1, R_Nq2/1
  Convert2/1 -> Mux6/2
  Convert1/1 -> Mux9/1, Relational2/1, R_Nq6/1, Logical2/1
  Relational/1 -> SWMaxi/1, Convert1/1, Mux5/1
  Convert4/1 -> Concat/2, Concat/1
  R_Nq6/1 -> Relational2/2
  R_Nq1/1 -> Mux9/2
  R_Nq/1 -> Convert5/1
  R_TraceBackStartHold/1 -> Mux2/2
  Const_0/1 -> SWMaxi/2
  Mux8/1 -> R_Nq1/1
  Relational2/1 -> R_Nq/1
  R_Nq2/1 -> Mux8/3, Mux7/2
  Const_1/1 -> Relational1/2
  Relational1/1 -> R_Nq3/1, Mux7/1, Mux8/1
  R_Nq5/1 -> Logical3/2
  R_Nq3/1 -> Mux6/1
  Logical1/1 -> R_Nq4/1, Logical2/2
  Concat/1 -> R_Nq5/1
  Subsystem/1(i(n)) -> R_NqE1/1
  Const_0_3/1 -> Mux7/3, Relational4/2
  Logical/1 -> Convert3/1
  R_Nq4/1 -> Logical1/2
  K_TraceBackStartHold/1 -> Mux2/3
  Logical2/1 -> Convert4/1
  "reset "/1 -> R_TraceBackStartHold/2
